simulink model "aie_firs_pl_multirate"  (R2023a)
settings: Solver=VariableStepAuto  StartTime=0.0  StopTime=0.0001  RelTol=1e-3
InitFcn:
  | SAMPLE_PERIOD_SEC=1/200E6;
undefined symbols (not defined in the file): None, S, vsva2197, xcvc1902, xlfda_numerator
libraries: hdlBasic x8, aieUtilities x2, aieDSP x2, dspsrcs4 x2, simulink x1, hdlUtilities x1, vmcUtilities x1
settings Model: Creator=abehbood  LastModifiedBy=robg
settings SolverCC: AlgebraicLoopSolver=TrustRegion
settings DebuggingCC: UnconnectedInputMsg=warning  UnconnectedOutputMsg=warning  UnconnectedLineMsg=warning
settings ModelReferenceCC: EnableRefExpFcnMdlSchedulingChecks=on
settings RTWCC: DLArmComputeVersion=19.05

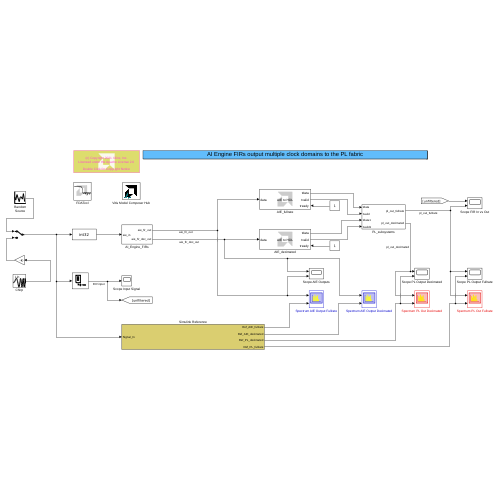
[thumbnail: Simulink's stored preview of the top-level diagram]
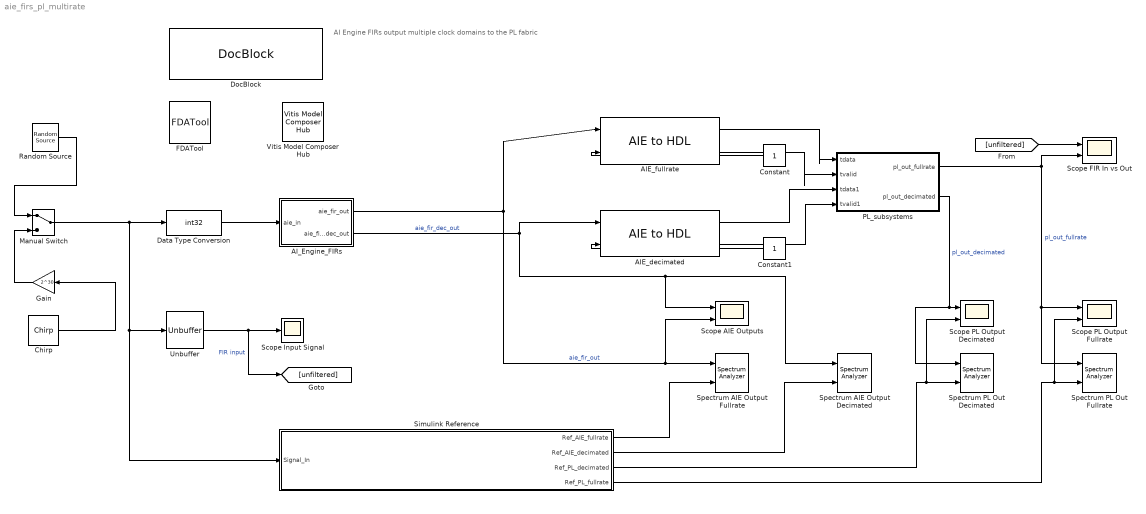
== system aie_firs_pl_multirate ==
  note: AI Engine FIRs output multiple clock domains to the PL fabric
  AIE_decimated : aieUtilities/AIE to HDL  OutDataType=int32  OutSampleTime=Inherit: Same as tready
  AIE_fullrate : aieUtilities/AIE to HDL  OutDataType=int32  OutSampleTime=Inherit: Same as tready
  AI_Engine_FIRs : Subsystem
  Chirp : dspsrcs4/Chirp  sweep=Linear  mode=Unidirectional  f0=1000  f1=50e6  t1=.0001  Tsweep=.0001  phase=0  Ts=1/200e6  spf=256  datatype=double  OutputFrames=off
  Constant : Constant  OutDataTypeStr=boolean
  Constant1 : Constant  OutDataTypeStr=boolean
  Data Type Conversion : DataTypeConversion  OutDataTypeStr=int32  SaturateOnIntegerOverflow=off  RndMeth=Floor
  DocBlock : simulink/Model-Wide Utilities/DocBlock  DocumentType=Text  mask(DocBlock){}
      content=|
      | ///////////////////////////////////////////////////////////////////////////
      | // Copyright 2023 Xilinx
      | //
      | // Licensed under the Apache License, Version 2.0 (the "License");
      | // you may not use this file except in compliance with the License.
      | // You may obtain a copy of the License at
      | //
      | // http://www.apache.org/licenses/LICENSE-2.0
      | //
      | // Unless required by applicable law or agreed to in writing, software
      | // distributed under the License is distributed on an "AS IS" BASIS,
      | // WITHOUT WARRANTIES OR CONDITIONS OF ANY KIND, either express or implied.
      | // See the License for the specific language governing permissions and
      | // limitations under the License.
      | ///////////////////////////////////////////////////////////////////////////
      mask Display:
      | xmcDrawBlockIcon();
      | disp(['{\fontsize{10pt}(c) Copyright 2021' ' Xilinx, Inc.}\newline \newline '],'texmode','on');
      | disp('{\fontsize{10pt}Licensed under the Apache License 2.0}','texmode','on');
      | disp('\newline \newline \newline{\fontsize{10pt}Double Click for Copyright Notice}','texmode','on');
  FDATool : hdlUtilities/FDATool  block_type=fdatool
      settings: infoedit=FDATool
  Gain : Gain  Gain=2^30
  Manual Switch : ManualSwitch
  PL_subsystems : Subsystem
  Random Source : dspsrcs4/Random Source  SrcType=Gaussian  NormMethod=Ziggurat  CltLength=12  MinVal=0  MaxVal=1  MeanVal=0  VarVal=2^30  RepMode=Not repeatable  rawSeed=1  IsInherit=off  SampMode=Discrete  SampTime=1/200e6  SampFrame=256  DataType=Double  OutComplex=Real  OutputFrames=off
  Scope AIE Outputs : Scope  NumInputPorts=2
  Scope FIR In vs Out : Scope  NumInputPorts=2
  Scope Input Signal : Scope
  Scope PL Output Decimated : Scope  NumInputPorts=2
  Scope PL Output Fullrate : Scope  NumInputPorts=2
  Simulink Reference : Subsystem
  Spectrum AIE Output Decimated : SpectrumAnalyzer  NumInputPorts=2  WindowPosition=[960 33 796 446]  Visible=on  SampleRate=100000000  PlotAsTwoSidedSpectrum=off  Span=50000000  CenterFrequency=25000000  StartFrequency=0  StopFrequency=50000000  AveragingMethod=Exponential  YLimits=[-53.8646,54.5647]  ShowLegend=on  ChannelNames="[\"\"]"  DefaultConfigurationName=spbscopes.SpectrumAnalyzerBlockCfg
      settings: OpenAtSimulationStart=off
  Spectrum AIE Output Fullrate : SpectrumAnalyzer  NumInputPorts=2  WindowPosition=[562 317 796 446]  Visible=on  SampleRate=200000000  PlotAsTwoSidedSpectrum=off  Span=100000000  CenterFrequency=50000000  StartFrequency=0  StopFrequency=100000000  AveragingMethod=Exponential  YLimits=[-30.2073,104.1879]  ShowLegend=on  ChannelNames="[\"\"]"  DefaultConfigurationName=spbscopes.SpectrumAnalyzerBlockCfg
      settings: OpenAtSimulationStart=off
  Spectrum PL Out Decimated : SpectrumAnalyzer  NumInputPorts=2  WindowPosition=[559 318 802 444]  Visible=on  SampleRate=100000000  PlotAsTwoSidedSpectrum=off  Span=50000000  CenterFrequency=25000000  StartFrequency=0  StopFrequency=50000000  AveragingMethod=Exponential  YLimits=[-54.0931,54.532]  ShowLegend=on  ChannelNames="[\"\"]"  DefaultConfigurationName=spbscopes.SpectrumAnalyzerBlockCfg
      settings: OpenAtSimulationStart=off
  Spectrum PL Out Fullrate : SpectrumAnalyzer  NumInputPorts=2  WindowPosition=[565 320 790 440]  Visible=on  SampleRate=200000000  PlotAsTwoSidedSpectrum=off  AxesScaling=Manual  Span=100000000  CenterFrequency=50000000  StartFrequency=0  StopFrequency=100000000  AveragingMethod=Exponential  YLimits=[-31.9987,103.7104]  ShowLegend=on  ChannelNames="[\"\"]"  DefaultConfigurationName=spbscopes.SpectrumAnalyzerBlockCfg
  Unbuffer : Unbuffer
  Vitis Model Composer Hub : vmcUtilities/Vitis Model Composer Hub  Tag=genX  CodeGeneration=off  StartColumn=1  NumberOfColumns=1  TargetDirectory=./code  exportDesign=off  analyzeDesign=off  validateDesignOnHw=off  ExportType=AI Engines  IpVendor=xilinx.com  IpLibrary=hls  IpVersion=1.0  IpHWLanguage=Verilog  AieCompilerOptions={}  AieSimulatorOptions={}  CreateTestbench=off  TestbenchStackSize=10  RunRtlSim=off  RunCSim=off  RunAieSim=off  AieSimTimeout=50000  RunAieSimProfiling=off  LaunchVitisAnalyzer=off  PlotOutput=off  RunX86Sim=off  X86SimTimeout=10  GenHwImage=off  GenLibadfXo=off  GenHwValidationCode=off  PlatformType=Not Specified  HwSystemType=Baremetal  HwValidationTarget=hw  ProjDevice=xcvc1902-vsva2197-1LP-e-S  ProjDevicePart=xcvc1902-vsva2197-1LP-e-S  AIEType=AIE  SamplePeriod=-1  ClockFrequency=200  DataPathParallelism=1  xilinxfamily=versalaicore  part=xcvc1902  speed=-1LP-e-S  package=vsva2197  directory=./netlist  testbench=off  incr_netlist=off  synthesis_tool=Vivado  clock_wrapper=Clock Enables  dbl_ovrd=According to Block Masks  dcm_input_clock_period=10  sysclk_period=10  simulink_period=1  eval_field=0  LogFileName=''  NThreads=4
  wires:
  Data Type Conversion/1 -> AI_Engine_FIRs/1(aie_in)
  AI_Engine_FIRs/1(aie_fir_out) -> Scope AIE Outputs/2, Spectrum AIE Output Fullrate/1, AIE_fullrate/1  "aie_fir_out"
  Constant/1 -> AIE_fullrate/2
  Simulink Reference/1(Ref_AIE_fullrate) -> Spectrum AIE Output Fullrate/2
  Simulink Reference/2(Ref_AIE_decimated) -> Spectrum AIE Output Decimated/2
  Simulink Reference/3(Ref_PL_decimated) -> Spectrum PL Out Decimated/2, Scope PL Output Decimated/2
  Simulink Reference/4(Ref_PL_fullrate) -> Scope PL Output Fullrate/2, Spectrum PL Out Fullrate/2
  Constant1/1 -> AIE_decimated/2
  AI_Engine_FIRs/2(aie_fir_dec_out) -> Scope AIE Outputs/1, Spectrum AIE Output Decimated/1, AIE_decimated/1  "aie_fir_dec_out"
  AIE_fullrate/1 -> PL_subsystems/1(tdata)
  AIE_fullrate/2 -> PL_subsystems/2(tvalid)
  AIE_decimated/1 -> PL_subsystems/3(tdata1)
  AIE_decimated/2 -> PL_subsystems/4(tvalid1)
  PL_subsystems/2(pl_out_decimated) -> Spectrum PL Out Decimated/1, Scope PL Output Decimated/1  "pl_out_decimated"
  PL_subsystems/1(pl_out_fullrate) -> Scope FIR In vs Out/2, Spectrum PL Out Fullrate/1, Scope PL Output Fullrate/1  "pl_out_fullrate"
  Manual Switch/1 -> Unbuffer/1, Simulink Reference/1(Signal_In), Data Type Conversion/1
  Chirp/1 -> Gain/1
  Gain/1 -> Manual Switch/2
  Random Source/1 -> Manual Switch/1
  Unbuffer/1 -> [unfiltered], Scope Input Signal/1  "FIR input"
  [unfiltered] -> Scope FIR In vs Out/1

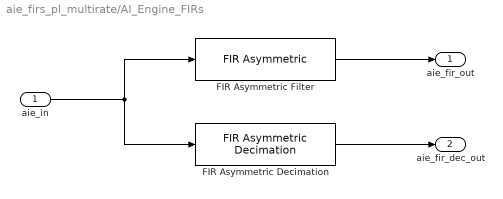
== system aie_firs_pl_multirate/AI_Engine_FIRs ==
  aie_in : Inport
  FIR Asymmetric Decimation : aieDSP/FIR Asymmetric Decimation  data_type=int32  coef_type=int32  use_coeff_reload=off  num_outputs=off  coeff=int32(xlfda_numerator(strcat(bdroot,'/FDATool'))*2^16)  fir_length=32  decimate_factor=2  input_window_size=256  shift_val=16  rnd_mode=Round to positive infinity  sat_mode=0-None  deci_poly=1  casc_length=1  AIE_VARIANT=1  blockJsonConstraints=[]  blockJsonConstraintsInternal=[]  spec=vmc_fir_decimate_asym.json  SerializedMaskParamNames=[]  SerializedMaskParamValues=[]  SerializedMaskParamVisibilities=[]  block_type=FIR Asymmetric Decimation  SerializedMaskParamDataypes=typename|typename|bool|bool|coef_type|uint|uint|uint|uint|uint|uint|uint|uint|uint  SerializedMaskParamEnumStrArr=0|0|0|0|0|0|0|0|0|Floor,Ceiling,Round to positive infinity,Round to negative infinity,Round symmetrical to infinity,Round symmetrical to zero,Round convergent to even,Round convergent to odd|0-None,1-Asymmetric,3-Symmetric|0|0|0  SerializedMaskParamEnumValArr=0|0|0|0|0|0|0|0|0|0,1,2,3,4,5,6,7|0,1,3|0|0|0  SerializedMaskParamVectorArr=0|0|0|0|1|0|0|0|0|0|0|0|0|0
  FIR Asymmetric Filter : aieDSP/FIR Asymmetric  data_type=int32  coef_type=int32  use_coeff_reload=off  num_outputs=off  coeff=int32(xlfda_numerator(strcat(bdroot,'/FDATool'))*2^16)  fir_length=32  input_window_size=256  shift_val=16  rnd_mode=Round to positive infinity  sat_mode=0-None  casc_length=1  AIE_VARIANT=1  blockJsonConstraints=[]  blockJsonConstraintsInternal=[]  spec=vmc_fir_sr_asym.json  SerializedMaskParamNames=[]  SerializedMaskParamValues=[]  SerializedMaskParamVisibilities=[]  block_type=FIR Asymmetric  SerializedMaskParamDataypes=typename|typename|bool|bool|coef_type|uint|uint|uint|uint|uint|uint|uint  SerializedMaskParamEnumStrArr=0|0|0|0|0|0|0|0|Floor,Ceiling,Round to positive infinity,Round to negative infinity,Round symmetrical to infinity,Round symmetrical to zero,Round convergent to even,Round convergent to odd|0-None,1-Asymmetric,3-Symmetric|0|0  SerializedMaskParamEnumValArr=0|0|0|0|0|0|0|0|0,1,2,3,4,5,6,7|0,1,3|0|0  SerializedMaskParamVectorArr=0|0|0|0|1|0|0|0|0|0|0|0
  aie_fir_out : Outport
  aie_fir_dec_out : Outport  Port=2
  wires:
  aie_in/1 -> FIR Asymmetric Filter/1, FIR Asymmetric Decimation/1
  FIR Asymmetric Filter/1 -> aie_fir_out/1
  FIR Asymmetric Decimation/1 -> aie_fir_dec_out/1

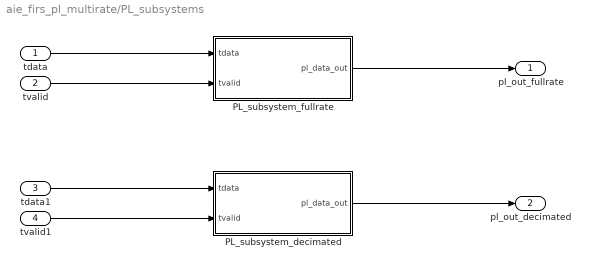
== system aie_firs_pl_multirate/PL_subsystems ==
  tdata : Inport
  tvalid : Inport  Port=2
  tdata1 : Inport  Port=3
  tvalid1 : Inport  Port=4
  PL_subsystem_decimated : Subsystem
  PL_subsystem_fullrate : Subsystem
  pl_out_fullrate : Outport
  pl_out_decimated : Outport  Port=2
  wires:
  tvalid1/1 -> PL_subsystem_decimated/2(tvalid)
  tdata/1 -> PL_subsystem_fullrate/1(tdata)
  tdata1/1 -> PL_subsystem_decimated/1(tdata)
  PL_subsystem_fullrate/1(pl_data_out) -> pl_out_fullrate/1
  PL_subsystem_decimated/1(pl_data_out) -> pl_out_decimated/1
  tvalid/1 -> PL_subsystem_fullrate/2(tvalid)

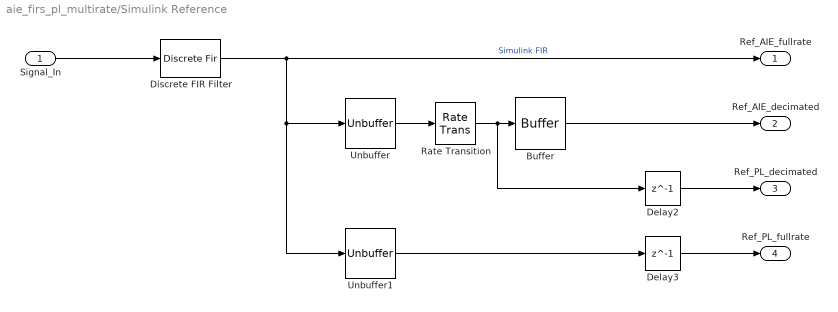
== system aie_firs_pl_multirate/Simulink Reference ==
  Signal_In : Inport
  Buffer : Buffer  N=128  OutputFrames=off
  Delay2 : Delay  DelayLength=1
  Delay3 : Delay  DelayLength=1
  Discrete FIR Filter : DiscreteFir  Coefficients=xlfda_numerator(strcat(bdroot,'/FDATool'))  InputProcessing=Columns as channels (frame based)  OutDataTypeStr=Inherit: Same as input
  Rate Transition : RateTransition  OutPortSampleTimeMultiple=1/2  OutPortSampleTime=1/100e6
  Unbuffer : Unbuffer
  Unbuffer1 : Unbuffer
  Ref_AIE_fullrate : Outport
  Ref_AIE_decimated : Outport  Port=2
  Ref_PL_decimated : Outport  Port=3
  Ref_PL_fullrate : Outport  Port=4
  wires:
  Rate Transition/1 -> Delay2/1, Buffer/1
  Discrete FIR Filter/1 -> Ref_AIE_fullrate/1, Unbuffer1/1, Unbuffer/1  "Simulink FIR"
  Signal_In/1 -> Discrete FIR Filter/1
  Unbuffer/1 -> Rate Transition/1
  Unbuffer1/1 -> Delay3/1
  Buffer/1 -> Ref_AIE_decimated/1
  Delay2/1 -> Ref_PL_decimated/1
  Delay3/1 -> Ref_PL_fullrate/1

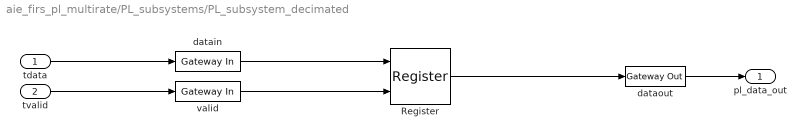
== system aie_firs_pl_multirate/PL_subsystems/PL_subsystem_decimated ==
  tdata : Inport
  tvalid : Inport  Port=2
  Register : hdlBasic/Register  init=0  rst=off  en=on  XmcBlockStatus=1  maskContainerNames=tabcontainer1  block_type=register  block_config=sysgen:Register_config
  datain : hdlBasic/Gateway In  gui_display_data_type=Fixed-point  arith_type=Signed (2's comp)  n_bits=32  bin_pt=0  preci_type=Single  exp_width=8  frac_width=24  rows=1  columns=1  quantization="Round  (unbiased: +/- Inf)"  overflow=Saturate  period=1/100e6  UseAsADC=off  ADCChannel='1'  interface=None  automatic_assignment=on  address_offset=hex2dec('00')  intf_name=''  intf_description=''  default_value=0  timing_constraint=None  locs_specified=off  LOCs={}  io_standard={}  inherit_from_input=off  hdl_port=on  XmcBlockStatus=1  maskContainerNames=group4  block_type=gatewayin  block_config=sysgen:gateway_in_config  block_width_w=590  block_height_w=620  block_width=640  block_height=850
  dataout : hdlBasic/Gateway Out  inherit_from_input=on  hdl_port=on  rows=1  columns=1  UseAsDAC=off  DACChannel='1'  interface=None  automatic_assignment=on  address_offset=hex2dec('00')  intf_name=''  intf_description=''  timing_constraint=None  locs_specified=off  LOCs={}  io_standard={}  XmcBlockStatus=1  maskContainerNames=group4  block_type=gatewayout  block_config=sysgen:gateway_out_config  block_width_w=590  block_height_w=620  block_width=620  block_height=750
  valid : hdlBasic/Gateway In  gui_display_data_type=Boolean  arith_type=Boolean  n_bits=16  bin_pt=14  preci_type=Single  exp_width=8  frac_width=24  rows=1  columns=1  quantization="Round  (unbiased: +/- Inf)"  overflow=Saturate  period=1/100e6  UseAsADC=off  ADCChannel='1'  interface=None  automatic_assignment=on  address_offset=hex2dec('00')  intf_name=''  intf_description=''  default_value=0  timing_constraint=None  locs_specified=off  LOCs={}  io_standard={}  inherit_from_input=off  hdl_port=on  XmcBlockStatus=1  maskContainerNames=group4  block_type=gatewayin  block_config=sysgen:gateway_in_config  block_width_w=590  block_height_w=620  block_width=640  block_height=850
  pl_data_out : Outport
  wires:
  valid/1 -> Register/2
  Register/1 -> dataout/1
  datain/1 -> Register/1
  tvalid/1 -> valid/1
  dataout/1 -> pl_data_out/1
  tdata/1 -> datain/1

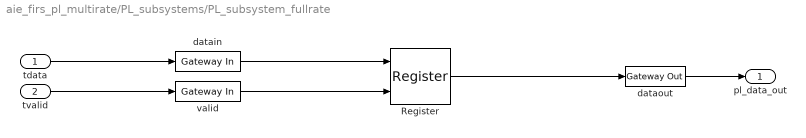
== system aie_firs_pl_multirate/PL_subsystems/PL_subsystem_fullrate ==
  tdata : Inport
  tvalid : Inport  Port=2
  Register : hdlBasic/Register  init=0  rst=off  en=on  XmcBlockStatus=1  maskContainerNames=tabcontainer1  block_type=register  block_config=sysgen:Register_config
  datain : hdlBasic/Gateway In  gui_display_data_type=Fixed-point  arith_type=Signed (2's comp)  n_bits=32  bin_pt=0  preci_type=Single  exp_width=8  frac_width=24  rows=1  columns=1  quantization="Round  (unbiased: +/- Inf)"  overflow=Saturate  period=1/200e6  UseAsADC=off  ADCChannel='1'  interface=None  automatic_assignment=on  address_offset=hex2dec('00')  intf_name=''  intf_description=''  default_value=0  timing_constraint=None  locs_specified=off  LOCs={}  io_standard={}  inherit_from_input=off  hdl_port=on  XmcBlockStatus=1  maskContainerNames=group4  block_type=gatewayin  block_config=sysgen:gateway_in_config  block_width_w=590  block_height_w=620  block_width=640  block_height=850
  dataout : hdlBasic/Gateway Out  inherit_from_input=on  hdl_port=on  rows=1  columns=1  UseAsDAC=off  DACChannel='1'  interface=None  automatic_assignment=on  address_offset=hex2dec('00')  intf_name=''  intf_description=''  timing_constraint=None  locs_specified=off  LOCs={}  io_standard={}  XmcBlockStatus=1  maskContainerNames=group4  block_type=gatewayout  block_config=sysgen:gateway_out_config  block_width_w=590  block_height_w=620  block_width=620  block_height=750
  valid : hdlBasic/Gateway In  gui_display_data_type=Boolean  arith_type=Boolean  n_bits=16  bin_pt=14  preci_type=Single  exp_width=8  frac_width=24  rows=1  columns=1  quantization="Round  (unbiased: +/- Inf)"  overflow=Saturate  period=1/200e6  UseAsADC=off  ADCChannel='1'  interface=None  automatic_assignment=on  address_offset=hex2dec('00')  intf_name=''  intf_description=''  default_value=0  timing_constraint=None  locs_specified=off  LOCs={}  io_standard={}  inherit_from_input=off  hdl_port=on  XmcBlockStatus=1  maskContainerNames=group4  block_type=gatewayin  block_config=sysgen:gateway_in_config  block_width_w=590  block_height_w=620  block_width=640  block_height=850
  pl_data_out : Outport
  wires:
  tdata/1 -> datain/1
  dataout/1 -> pl_data_out/1
  tvalid/1 -> valid/1
  datain/1 -> Register/1
  Register/1 -> dataout/1
  valid/1 -> Register/2
